simulink model "MOT_CTRL_MOT_FUN_001"  (R2025a)
settings: Solver=FixedStepAuto  StartTime=0.0  StopTime=10  FixedStep=1e-4  RelTol=1e-3
libraries: simulink x1
settings Model: DataDictionary=DcMotor.sldd  Creator=tecnicomcbti  LastModifiedBy=tecnicomcbti
settings SolverCC: ConcurrentTasks=on  PositivePriorityOrder=on
settings OptimizationCC: BlockReduction=off  OptimizeBlockIOStorage=off  ZeroExternalMemoryAtStartup=off  ZeroInternalMemoryAtStartup=off
settings DebuggingCC: AlgebraicLoopMsg=none  TasksWithSamePriorityMsg=none
settings RTWCC: Toolchain=Simulink Real-Time Toolchain  BuildConfiguration=Faster Runs  CodeExecutionProfiling=on  TargetLang=C++
settings GRTTargetCC: TargetLangStandard=C++03 (ISO)  CodeInterfacePackaging=C++ class  SubcomponentCodeInterfacePackaging=C++ class

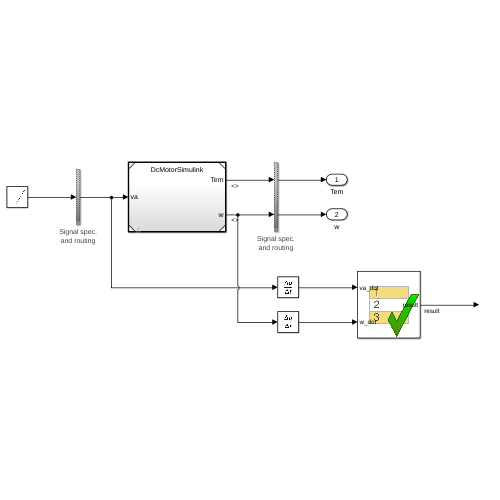
[thumbnail: Simulink's stored preview of the top-level diagram]
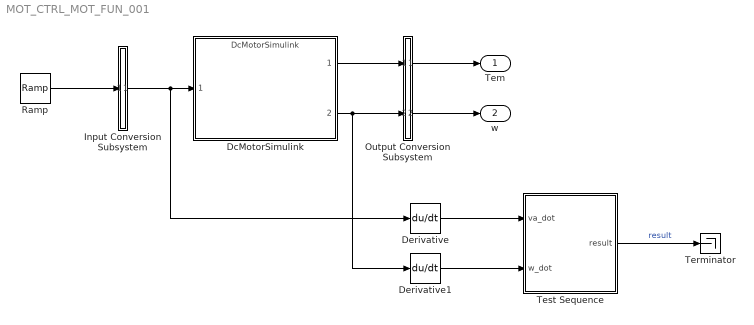
== system MOT_CTRL_MOT_FUN_001 ==
  DcMotorSimulink : ModelReference  ModelNameDialog=DcMotorSimulink  SimulationMode=Normal  ModelReferenceVersion=2.8
  Derivative : Derivative
  Derivative1 : Derivative
  Input Conversion Subsystem : Subsystem  Tag=__SLT_ICS__  Description=|
      | Signal spec.
      | and routing
      settings: AttributesFormatString=%<Description>
  Output Conversion Subsystem : Subsystem  Tag=__SLT_OCS__  Description=|
      | Signal spec.
      | and routing
      settings: AttributesFormatString=%<Description>
  Ramp : simulink/Sources/Ramp  slope=33  start=0  InitialOutput=0
  Terminator : Terminator
  Test Sequence : Test Sequence  TreatAsAtomicUnit=on
  Tem : Outport
  w : Outport  Port=2
  wires:
  Output Conversion Subsystem/1(Outport_1) -> Tem/1
  Output Conversion Subsystem/2(Outport_2) -> w/1
  Input Conversion Subsystem/1(Outport_1) -> Derivative/1, DcMotorSimulink/1
  DcMotorSimulink/1 -> Output Conversion Subsystem/1(Inport_1)
  DcMotorSimulink/2 -> Derivative1/1, Output Conversion Subsystem/2(Inport_2)
  Test Sequence/1(result) -> Terminator/1  "result"
  Derivative/1 -> Test Sequence/1(va_dot)
  Derivative1/1 -> Test Sequence/2(w_dot)
  Ramp/1 -> Input Conversion Subsystem/1(Inport_1)

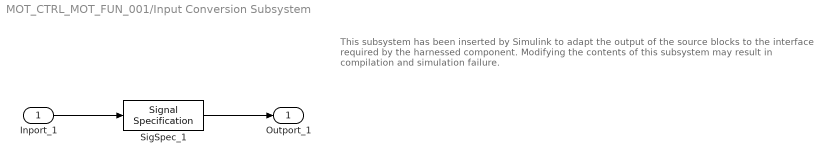
== system MOT_CTRL_MOT_FUN_001/Input Conversion Subsystem ==
  note: This subsystem has been inserted by Simulink to adapt the output of the source blocks to the interface required by the harnessed component.
      |  Modifying the contents of this subsystem may result in compilation and simulation failure.
  Inport_1 : Inport
  SigSpec_1 : SignalSpecification  OutDataTypeStr=double  Dimensions=[1]  SampleTime=[0, 0]
  Outport_1 : Outport
  wires:
  SigSpec_1/1 -> Outport_1/1
  Inport_1/1 -> SigSpec_1/1

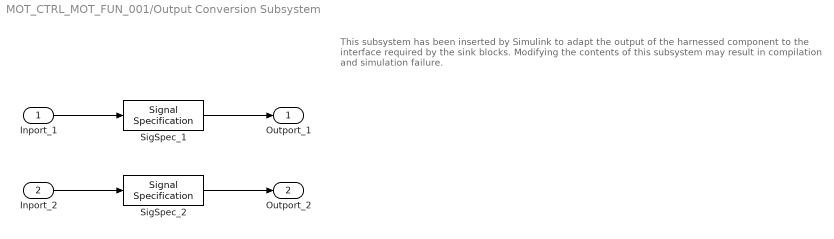
== system MOT_CTRL_MOT_FUN_001/Output Conversion Subsystem ==
  note: This subsystem has been inserted by Simulink to adapt the output of the harnessed component to the interface required by the sink blocks.
      |  Modifying the contents of this subsystem may result in compilation and simulation failure.
  Inport_1 : Inport
  Inport_2 : Inport  Port=2
  SigSpec_1 : SignalSpecification  OutDataTypeStr=double  Dimensions=[1]
  SigSpec_2 : SignalSpecification  OutDataTypeStr=double  Dimensions=[1]
  Outport_1 : Outport
  Outport_2 : Outport  Port=2
  wires:
  Inport_1/1 -> SigSpec_1/1
  SigSpec_1/1 -> Outport_1/1
  Inport_2/1 -> SigSpec_2/1
  SigSpec_2/1 -> Outport_2/1

== stateflow chart MOT_CTRL_MOT_FUN_001/Test Sequence ==
  state Idle
  state Comparasion
    if((va_dot > 0) && (w_dot > 0))
    result = true;
    else
    result = false;
    end
  (default) -> Idle
  Idle -> Comparasion : [
      | after(1e-4, sec)
      | ]
  data: va_dot input; w_dot input; result output
